simulink model "Model"  (R2020b)
settings: Solver=FixedStepAuto  StartTime=0.0  StopTime=12250  FixedStep=0.05  RelTol=1e-3
libraries: simulink x4
settings Model: Creator=Damerius  LastModifiedBy=Scythe
settings DataIOCC: ReturnWorkspaceOutputs=off
settings DebuggingCC: InheritedTsInSrcMsg=none  ArithmeticOperatorsInVariantConditions=warning
settings SFSimCC: SimUseLocalCustomCode=off  CustomCodeUndefinedFunction=UseInterfaceOnly
settings RTWCC: RTWUseLocalCustomCode=off

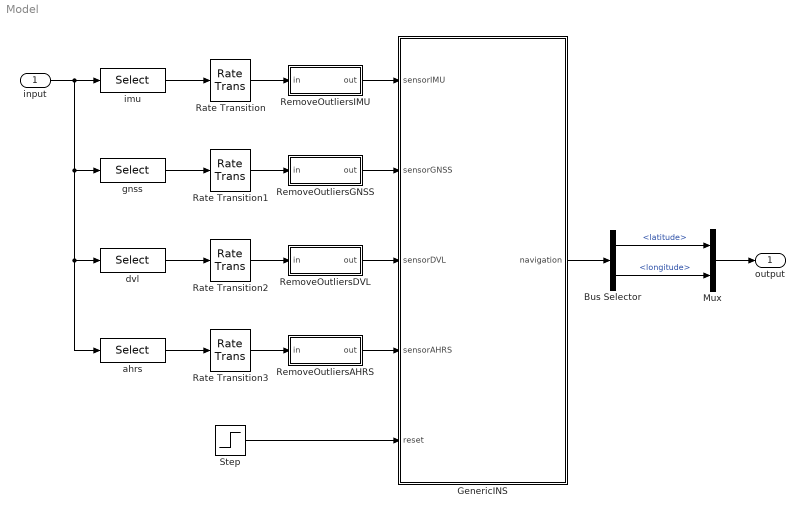
== system Model ==
  input : Inport
  Bus Selector : BusSelector  OutputSignals=latitude,longitude
  GenericINS : Subsystem
  Mux : Mux  Inputs=2
  Rate Transition{,1..3} (4 alike) : RateTransition  Integrity=off  Deterministic=off  OutPortSampleTime=0.05
  RemoveOutliersAHRS : Subsystem
  RemoveOutliersDVL : Subsystem
  RemoveOutliersGNSS : Subsystem
  RemoveOutliersIMU : Subsystem
  Step : Step  Time=0.05  Before=1  After=0
  ahrs : Selector  InputPortWidth=19  IndexOptions=Index vector (dialog)  Indices=16:19  OutputSizes=1
  dvl : Selector  InputPortWidth=19  IndexOptions=Index vector (dialog)  Indices=12:15  OutputSizes=1
  gnss : Selector  InputPortWidth=19  IndexOptions=Index vector (dialog)  Indices=8:11  OutputSizes=1
  imu : Selector  InputPortWidth=19  IndexOptions=Index vector (dialog)  Indices=1:7  OutputSizes=1
  output : Outport  VectorParamsAs1DForOutWhenUnconnected=off
  wires:
  input/1 -> imu/1, ahrs/1, dvl/1, gnss/1
  Mux/1 -> output/1
  Rate Transition1/1 -> RemoveOutliersGNSS/1(in)
  Rate Transition2/1 -> RemoveOutliersDVL/1(in)
  Rate Transition3/1 -> RemoveOutliersAHRS/1(in)
  imu/1 -> Rate Transition/1
  gnss/1 -> Rate Transition1/1
  dvl/1 -> Rate Transition2/1
  ahrs/1 -> Rate Transition3/1
  Rate Transition/1 -> RemoveOutliersIMU/1(in)
  RemoveOutliersIMU/1(out) -> GenericINS/1(sensorIMU)
  RemoveOutliersGNSS/1(out) -> GenericINS/2(sensorGNSS)
  RemoveOutliersDVL/1(out) -> GenericINS/3(sensorDVL)
  RemoveOutliersAHRS/1(out) -> GenericINS/4(sensorAHRS)
  GenericINS/1(navigation) -> Bus Selector/1
  Bus Selector/2 -> Mux/2  "<longitude>"
  Bus Selector/1 -> Mux/1  "<latitude>"
  Step/1 -> GenericINS/5(reset)

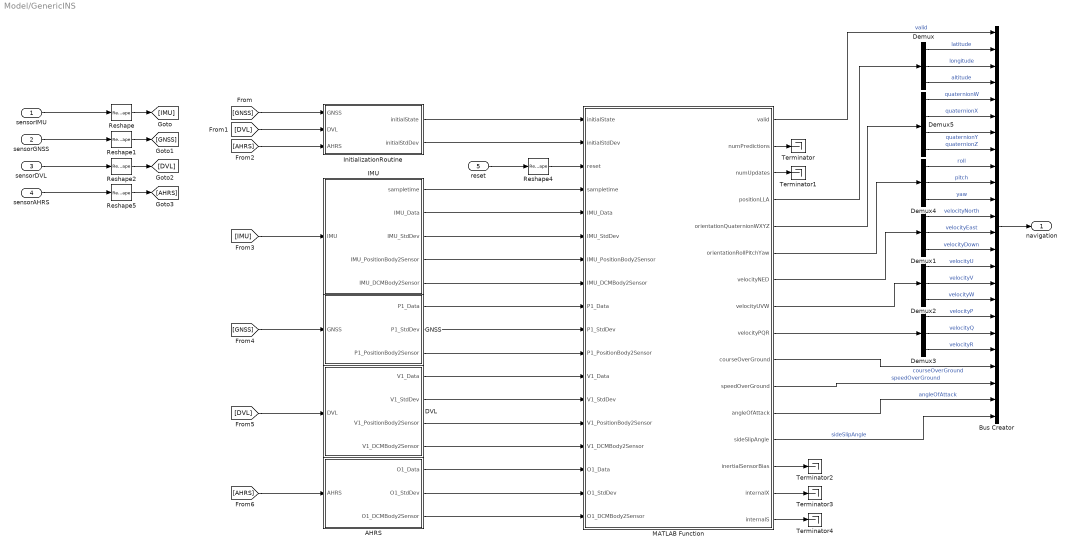
== system Model/GenericINS ==
  sensorIMU : Inport
  sensorGNSS : Inport  Port=2
  sensorDVL : Inport  Port=3
  sensorAHRS : Inport  Port=4
  reset : Inport  Port=5
  AHRS : Subsystem
  Bus Creator : BusCreator  Inputs=24
  DVL : Subsystem
  Demux{,1..4} (5 alike) : Demux  Outputs=3
  Demux5 : Demux
  GNSS : Subsystem
  IMU : Subsystem
  InitializationRoutine : Subsystem
  MATLAB Function : MATLAB Function  TreatAsAtomicUnit=on
  Reshape : Reshape  OutputDimensionality=Customize  OutputDimensions=[7,1]
  Reshape1 : Reshape  OutputDimensionality=Customize  OutputDimensions=[4,1]
  Reshape2 : Reshape  OutputDimensionality=Customize  OutputDimensions=[4,1]
  Reshape4 : Reshape  OutputDimensionality=Customize
  Reshape5 : Reshape  OutputDimensionality=Customize  OutputDimensions=[4,1]
  Terminator{,1..4} (5 alike) : Terminator
  navigation : Outport  VectorParamsAs1DForOutWhenUnconnected=off
  wires:
  Reshape5/1 -> [AHRS]
  sensorAHRS/1 -> Reshape5/1
  Reshape4/1 -> MATLAB Function/3(reset)
  reset/1 -> Reshape4/1
  Reshape2/1 -> [DVL]
  Reshape1/1 -> [GNSS]
  Reshape/1 -> [IMU]
  sensorGNSS/1 -> Reshape1/1
  sensorDVL/1 -> Reshape2/1
  sensorIMU/1 -> Reshape/1
  MATLAB Function/4(positionLLA) -> Demux/1
  MATLAB Function/7(velocityNED) -> Demux1/1
  MATLAB Function/8(velocityUVW) -> Demux2/1
  MATLAB Function/9(velocityPQR) -> Demux3/1
  MATLAB Function/5(orientationQuaternionWXYZ) -> Demux5/1
  Demux/1 -> Bus Creator/2  "latitude"
  Demux/2 -> Bus Creator/3  "longitude"
  Demux/3 -> Bus Creator/4  "altitude"
  Demux5/1 -> Bus Creator/5  "quaternionW"
  Demux5/2 -> Bus Creator/6  "quaternionX"
  Demux5/3 -> Bus Creator/7  "quaternionY"
  Demux5/4 -> Bus Creator/8  "quaternionZ"
  Demux4/1 -> Bus Creator/9  "roll"
  Demux4/2 -> Bus Creator/10  "pitch"
  Demux4/3 -> Bus Creator/11  "yaw"
  Demux1/1 -> Bus Creator/12  "velocityNorth"
  Demux1/2 -> Bus Creator/13  "velocityEast"
  Demux1/3 -> Bus Creator/14  "velocityDown"
  Demux2/1 -> Bus Creator/15  "velocityU"
  Demux2/2 -> Bus Creator/16  "velocityV"
  Demux2/3 -> Bus Creator/17  "velocityW"
  Demux3/1 -> Bus Creator/18  "velocityP"
  Demux3/2 -> Bus Creator/19  "velocityQ"
  Demux3/3 -> Bus Creator/20  "velocityR"
  Bus Creator/1 -> navigation/1
  InitializationRoutine/1(initialState) -> MATLAB Function/1(initialState)
  InitializationRoutine/2(initialStdDev) -> MATLAB Function/2(initialStdDev)
  [GNSS] -> InitializationRoutine/1(GNSS)
  [DVL] -> InitializationRoutine/2(DVL)
  [AHRS] -> InitializationRoutine/3(AHRS)
  [IMU] -> IMU/1(IMU)
  IMU/1(sampletime) -> MATLAB Function/4(sampletime)
  IMU/2(IMU_Data) -> MATLAB Function/5(IMU_Data)
  IMU/4(IMU_PositionBody2Sensor) -> MATLAB Function/7(IMU_PositionBody2Sensor)
  IMU/5(IMU_DCMBody2Sensor) -> MATLAB Function/8(IMU_DCMBody2Sensor)
  GNSS/3(P1_PositionBody2Sensor) -> MATLAB Function/11(P1_PositionBody2Sensor)
  [GNSS] -> GNSS/1(GNSS)
  DVL/3(V1_PositionBody2Sensor) -> MATLAB Function/14(V1_PositionBody2Sensor)
  DVL/4(V1_DCMBody2Sensor) -> MATLAB Function/15(V1_DCMBody2Sensor)
  [DVL] -> DVL/1(DVL)
  AHRS/3(O1_DCMBody2Sensor) -> MATLAB Function/18(O1_DCMBody2Sensor)
  [AHRS] -> AHRS/1(AHRS)
  MATLAB Function/6(orientationRollPitchYaw) -> Demux4/1
  MATLAB Function/1(valid) -> Bus Creator/1  "valid"
  MATLAB Function/10(courseOverGround) -> Bus Creator/21  "courseOverGround"
  MATLAB Function/11(speedOverGround) -> Bus Creator/22  "speedOverGround"
  MATLAB Function/12(angleOfAttack) -> Bus Creator/23  "angleOfAttack"
  MATLAB Function/13(sideSlipAngle) -> Bus Creator/24  "sideSlipAngle"
  AHRS/1(O1_Data) -> MATLAB Function/16(O1_Data)
  AHRS/2(O1_StdDev) -> MATLAB Function/17(O1_StdDev)
  DVL/2(V1_StdDev) -> MATLAB Function/13(V1_StdDev)
  GNSS/1(P1_Data) -> MATLAB Function/9(P1_Data)
  GNSS/2(P1_StdDev) -> MATLAB Function/10(P1_StdDev)
  IMU/3(IMU_StdDev) -> MATLAB Function/6(IMU_StdDev)
  DVL/1(V1_Data) -> MATLAB Function/12(V1_Data)
  MATLAB Function/2(numPredictions) -> Terminator/1
  MATLAB Function/3(numUpdates) -> Terminator1/1
  MATLAB Function/14(inertialSensorBias) -> Terminator2/1
  MATLAB Function/15(internalX) -> Terminator3/1
  MATLAB Function/16(internalS) -> Terminator4/1

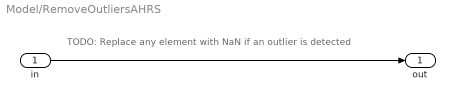
== system Model/RemoveOutliersAHRS ==
  note: TODO: Replace any element with NaN if an outlier is detected
  in : Inport
  out : Outport  VectorParamsAs1DForOutWhenUnconnected=off
  wires:
  in/1 -> out/1

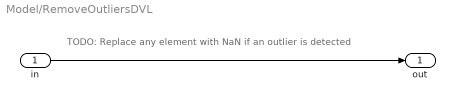
== system Model/RemoveOutliersDVL ==
  note: TODO: Replace any element with NaN if an outlier is detected
  in : Inport
  out : Outport  VectorParamsAs1DForOutWhenUnconnected=off
  wires:
  in/1 -> out/1

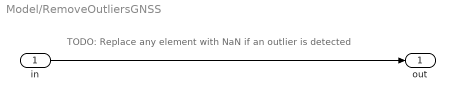
== system Model/RemoveOutliersGNSS ==
  note: TODO: Replace any element with NaN if an outlier is detected
  in : Inport
  out : Outport  VectorParamsAs1DForOutWhenUnconnected=off
  wires:
  in/1 -> out/1

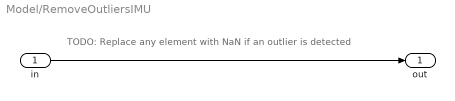
== system Model/RemoveOutliersIMU ==
  note: TODO: Replace any element with NaN if an outlier is detected
  in : Inport
  out : Outport  VectorParamsAs1DForOutWhenUnconnected=off
  wires:
  in/1 -> out/1

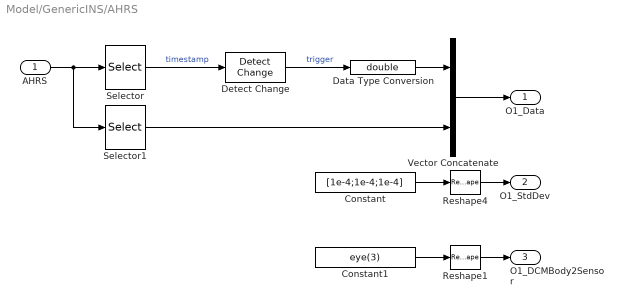
== system Model/GenericINS/AHRS ==
  AHRS : Inport
  Constant : Constant  Value=[1e-4;1e-4;1e-4]
  Constant1 : Constant  Value=eye(3)
  Data Type Conversion : DataTypeConversion  OutDataTypeStr=double
  Detect Change : simulink/Logic and Bit Operations/Detect Change  vinit=0  OutDataTypeStr=boolean
  Reshape1 : Reshape  OutputDimensionality=Customize  OutputDimensions=[3,3]
  Reshape4 : Reshape  OutputDimensionality=Customize  OutputDimensions=[3,1]
  Selector : Selector  InputPortWidth=4  IndexOptions=Index vector (dialog)  Indices=1  OutputSizes=1
  Selector1 : Selector  InputPortWidth=4  IndexOptions=Index vector (dialog)  Indices=2:4  OutputSizes=1
  Vector Concatenate : Concatenate
  O1_Data : Outport  VectorParamsAs1DForOutWhenUnconnected=off
  O1_StdDev : Outport  Port=2  VectorParamsAs1DForOutWhenUnconnected=off
  O1_DCMBody2Sensor : Outport  Port=3  VectorParamsAs1DForOutWhenUnconnected=off
  wires:
  Constant1/1 -> Reshape1/1
  Constant/1 -> Reshape4/1
  Vector Concatenate/1 -> O1_Data/1
  Selector1/1 -> Vector Concatenate/2
  Data Type Conversion/1 -> Vector Concatenate/1
  Detect Change/1 -> Data Type Conversion/1  "trigger"
  Selector/1 -> Detect Change/1  "timestamp"
  AHRS/1 -> Selector/1, Selector1/1
  Reshape4/1 -> O1_StdDev/1
  Reshape1/1 -> O1_DCMBody2Sensor/1

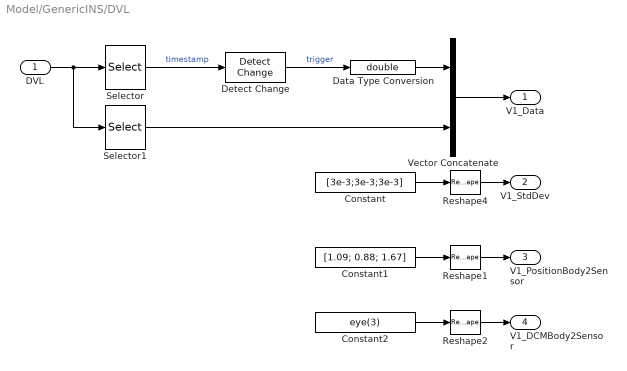
== system Model/GenericINS/DVL ==
  DVL : Inport
  Constant : Constant  Value=[3e-3;3e-3;3e-3]
  Constant1 : Constant  Value=[1.09; 0.88; 1.67]
  Constant2 : Constant  Value=eye(3)
  Data Type Conversion : DataTypeConversion  OutDataTypeStr=double
  Detect Change : simulink/Logic and Bit Operations/Detect Change  vinit=0  OutDataTypeStr=boolean
  Reshape1 : Reshape  OutputDimensionality=Customize  OutputDimensions=[3,1]
  Reshape2 : Reshape  OutputDimensionality=Customize  OutputDimensions=[3,3]
  Reshape4 : Reshape  OutputDimensionality=Customize  OutputDimensions=[3,1]
  Selector : Selector  InputPortWidth=4  IndexOptions=Index vector (dialog)  Indices=1  OutputSizes=1
  Selector1 : Selector  InputPortWidth=4  IndexOptions=Index vector (dialog)  Indices=2:4  OutputSizes=1
  Vector Concatenate : Concatenate
  V1_Data : Outport  VectorParamsAs1DForOutWhenUnconnected=off
  V1_StdDev : Outport  Port=2  VectorParamsAs1DForOutWhenUnconnected=off
  V1_PositionBody2Sensor : Outport  Port=3  VectorParamsAs1DForOutWhenUnconnected=off
  V1_DCMBody2Sensor : Outport  Port=4  VectorParamsAs1DForOutWhenUnconnected=off
  wires:
  Constant1/1 -> Reshape1/1
  Constant/1 -> Reshape4/1
  Vector Concatenate/1 -> V1_Data/1
  Selector1/1 -> Vector Concatenate/2
  Data Type Conversion/1 -> Vector Concatenate/1
  Detect Change/1 -> Data Type Conversion/1  "trigger"
  Selector/1 -> Detect Change/1  "timestamp"
  DVL/1 -> Selector/1, Selector1/1
  Constant2/1 -> Reshape2/1
  Reshape4/1 -> V1_StdDev/1
  Reshape1/1 -> V1_PositionBody2Sensor/1
  Reshape2/1 -> V1_DCMBody2Sensor/1

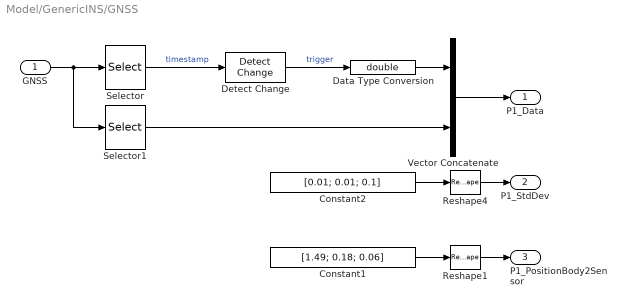
== system Model/GenericINS/GNSS ==
  GNSS : Inport
  Constant1 : Constant  Value=[1.49; 0.18; 0.06]
  Constant2 : Constant  Value=[0.01; 0.01; 0.1]
  Data Type Conversion : DataTypeConversion  OutDataTypeStr=double
  Detect Change : simulink/Logic and Bit Operations/Detect Change  vinit=0  OutDataTypeStr=boolean
  Reshape1 : Reshape  OutputDimensionality=Customize  OutputDimensions=[3,1]
  Reshape4 : Reshape  OutputDimensionality=Customize  OutputDimensions=[3,1]
  Selector : Selector  InputPortWidth=4  IndexOptions=Index vector (dialog)  Indices=1  OutputSizes=1
  Selector1 : Selector  InputPortWidth=4  IndexOptions=Index vector (dialog)  Indices=2:4  OutputSizes=1
  Vector Concatenate : Concatenate
  P1_Data : Outport  VectorParamsAs1DForOutWhenUnconnected=off
  P1_StdDev : Outport  Port=2  VectorParamsAs1DForOutWhenUnconnected=off
  P1_PositionBody2Sensor : Outport  Port=3  VectorParamsAs1DForOutWhenUnconnected=off
  wires:
  GNSS/1 -> Selector1/1, Selector/1
  Selector/1 -> Detect Change/1  "timestamp"
  Detect Change/1 -> Data Type Conversion/1  "trigger"
  Data Type Conversion/1 -> Vector Concatenate/1
  Selector1/1 -> Vector Concatenate/2
  Vector Concatenate/1 -> P1_Data/1
  Constant2/1 -> Reshape4/1
  Constant1/1 -> Reshape1/1
  Reshape4/1 -> P1_StdDev/1
  Reshape1/1 -> P1_PositionBody2Sensor/1

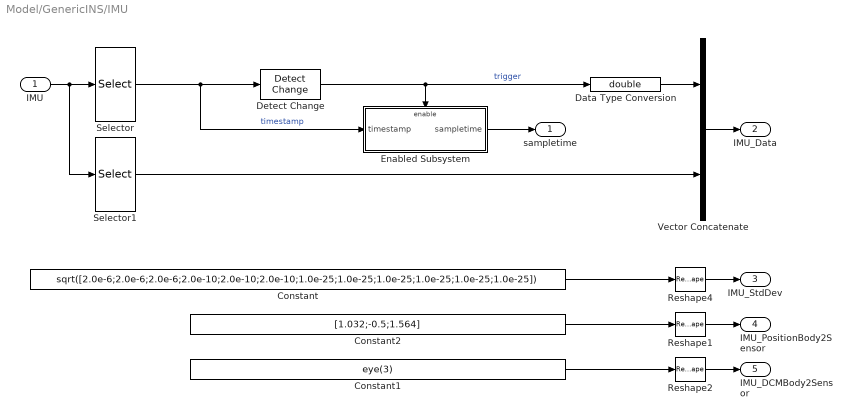
== system Model/GenericINS/IMU ==
  IMU : Inport
  Constant : Constant  Value=sqrt([2.0e-6;2.0e-6;2.0e-6;2.0e-10;2.0e-10;2.0e-10;1.0e-25;1.0e-25;1.0e-25;1.0e-25;1.0e-25;1.0e-25])
  Constant1 : Constant  Value=eye(3)
  Constant2 : Constant  Value=[1.032;-0.5;1.564]
  Data Type Conversion : DataTypeConversion  OutDataTypeStr=double
  Detect Change : simulink/Logic and Bit Operations/Detect Change  vinit=0  OutDataTypeStr=boolean
  Enabled Subsystem : Subsystem  TreatAsAtomicUnit=on
  Reshape1 : Reshape  OutputDimensionality=Customize  OutputDimensions=[3,1]
  Reshape2 : Reshape  OutputDimensionality=Customize  OutputDimensions=[3,3]
  Reshape4 : Reshape  OutputDimensionality=Customize  OutputDimensions=[12,1]
  Selector : Selector  InputPortWidth=7  IndexOptions=Index vector (dialog)  Indices=1  OutputSizes=1
  Selector1 : Selector  InputPortWidth=7  IndexOptions=Index vector (dialog)  Indices=2:7  OutputSizes=1
  Vector Concatenate : Concatenate
  sampletime : Outport  VectorParamsAs1DForOutWhenUnconnected=off
  IMU_Data : Outport  Port=2  VectorParamsAs1DForOutWhenUnconnected=off
  IMU_StdDev : Outport  Port=3  VectorParamsAs1DForOutWhenUnconnected=off
  IMU_PositionBody2Sensor : Outport  Port=4  VectorParamsAs1DForOutWhenUnconnected=off
  IMU_DCMBody2Sensor : Outport  Port=5  VectorParamsAs1DForOutWhenUnconnected=off
  wires:
  Constant/1 -> Reshape4/1
  Constant1/1 -> Reshape2/1
  Constant2/1 -> Reshape1/1
  Selector/1 -> Enabled Subsystem/1(timestamp), Detect Change/1  "timestamp"
  Detect Change/1 -> Enabled Subsystem/Enable, Data Type Conversion/1  "trigger"
  Enabled Subsystem/1(sampletime) -> sampletime/1
  Data Type Conversion/1 -> Vector Concatenate/1
  IMU/1 -> Selector1/1, Selector/1
  Selector1/1 -> Vector Concatenate/2
  Vector Concatenate/1 -> IMU_Data/1
  Reshape4/1 -> IMU_StdDev/1
  Reshape1/1 -> IMU_PositionBody2Sensor/1
  Reshape2/1 -> IMU_DCMBody2Sensor/1

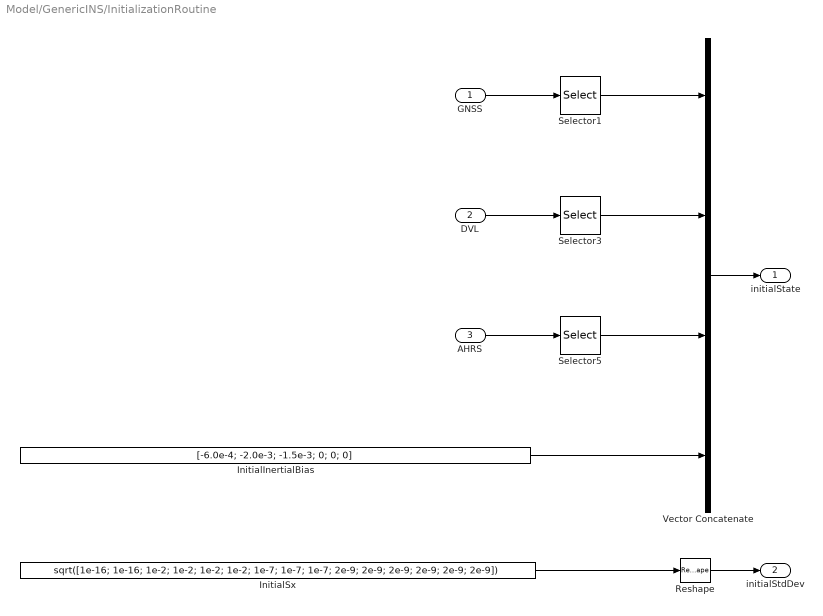
== system Model/GenericINS/InitializationRoutine ==
  GNSS : Inport
  DVL : Inport  Port=2
  AHRS : Inport  Port=3
  InitialInertialBias : Constant  Value=[-6.0e-4; -2.0e-3; -1.5e-3; 0; 0; 0]
  InitialSx : Constant  Value=sqrt([1e-16; 1e-16; 1e-2; 1e-2; 1e-2; 1e-2; 1e-7; 1e-7; 1e-7; 2e-9; 2e-9; 2e-9; 2e-9; 2e-9; 2e-9])
  Reshape : Reshape  OutputDimensionality=Customize  OutputDimensions=[15,1]
  Selector1 : Selector  InputPortWidth=4  IndexOptions=Index vector (dialog)  Indices=2:4  OutputSizes=1
  Selector3 : Selector  InputPortWidth=4  IndexOptions=Index vector (dialog)  Indices=2:4  OutputSizes=1
  Selector5 : Selector  InputPortWidth=4  IndexOptions=Index vector (dialog)  Indices=2:4  OutputSizes=1
  Vector Concatenate : Concatenate  NumInputs=4
  initialState : Outport  VectorParamsAs1DForOutWhenUnconnected=off
  initialStdDev : Outport  Port=2  VectorParamsAs1DForOutWhenUnconnected=off
  wires:
  Selector1/1 -> Vector Concatenate/1
  GNSS/1 -> Selector1/1
  DVL/1 -> Selector3/1
  Selector3/1 -> Vector Concatenate/2
  Selector5/1 -> Vector Concatenate/3
  AHRS/1 -> Selector5/1
  InitialInertialBias/1 -> Vector Concatenate/4
  Vector Concatenate/1 -> initialState/1
  Reshape/1 -> initialStdDev/1
  InitialSx/1 -> Reshape/1

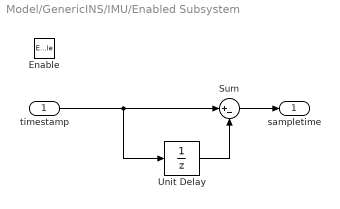
== system Model/GenericINS/IMU/Enabled Subsystem ==
  timestamp : Inport
  Enable : EnablePort
  Sum : Sum  Inputs=|+-
  Unit Delay : UnitDelay  SampleTime=-1  HasFrameUpgradeWarning=on
  sampletime : Outport  VectorParamsAs1DForOutWhenUnconnected=off
  wires:
  timestamp/1 -> Unit Delay/1, Sum/1
  Unit Delay/1 -> Sum/2
  Sum/1 -> sampletime/1

== matlab function Model/GenericINS/MATLAB Function ==
  data: initialState input; valid output; numPredictions output; numUpdates output; initialStdDev input; reset input; sampletime input; IMU_Data input; IMU_StdDev input; IMU_PositionBody2Sensor input; IMU_DCMBody2Sensor input; P1_Data input; P1_StdDev input; P1_PositionBody2Sensor input; V1_Data input; V1_StdDev input; V1_PositionBody2Sensor input; V1_DCMBody2Sensor input; O1_Data input; O1_StdDev input; O1_DCMBody2Sensor input; positionLLA output; orientationQuaternionWXYZ output; orientationRollPitchYaw output; velocityNED output; velocityUVW output; velocityPQR output; courseOverGround output; speedOverGround output; angleOfAttack output; sideSlipAngle output; inertialSensorBias output; internalX output; internalS output
function [valid, numPredictions, numUpdates, positionLLA, orientationQuaternionWXYZ, orientationRollPitchYaw, velocityNED, velocityUVW, velocityPQR, courseOverGround, speedOverGround, angleOfAttack, sideSlipAngle, inertialSensorBias, internalX, internalS] = ExampleINS(initialState, initialStdDev, reset, sampletime, IMU_Data, IMU_StdDev, IMU_PositionBody2Sensor, IMU_DCMBody2Sensor, P1_Data, P1_StdDev, P1_PositionBody2Sensor, V1_Data, V1_StdDev, V1_PositionBody2Sensor, V1_DCMBody2Sensor, O1_Data, O1_StdDev, O1_DCMBody2Sensor)
    %ExampleINS Generated MATLAB function for a generic inertial navigation system (1 position measurements, 1 velocity measurements, 1 orientation measurements).
    % This function was automatically generated using the command GenericINS.GenerateFunction('ExampleINS', [3], [3], [3], 0).
    % 
    % PARAMETERS
    % initialState               ... 15-by-1 initial state vector to be used when the INS is reset. The elements are as follows:
    %                                 1: latitude     [rad]     Initial latitude of the position of the IMU.
    %                                 2: longitude    [rad]     Initial longitude of the position of the IMU.
    %                                 3: altitude     [m]       Initial altitude of the position of the IMU, positive upwards.
    %                                 4: velocityU    [m/s]     Initial body-fixed velocity in x-direction of the body-frame at the position of the IMU.
    %                                 5: velocityV    [m/s]     Initial body-fixed velocity in y-direction of the body-frame at the position of the IMU.
    %                                 6: velocityW    [m/s]     Initial body-fixed velocity in z-direction of the body-frame at the position of the IMU.
    %                                 7: roll         [rad]     Initial roll angle.
    %                                 8: pitch        [rad]     Initial pitch angle.
    %                                 9: yaw          [rad]     Initial yaw angle.
    %                                10: biasAccX     [m/(s*s)] Initial acceleration bias in x-direction of IMU sensor frame.
    %                                11: biasAccY     [m/(s*s)] Initial acceleration bias in y-direction of IMU sensor frame.
    %                                12: biasAccZ     [m/(s*s)] Initial acceleration bias in z-direction of IMU sensor frame.
    %                                13: biasGyrX     [rad/s]   Initial angular rate bias around x-axis of IMU sensor frame.
    %                                14: biasGyrY     [rad/s]   Initial angular rate bias around y-axis of IMU sensor frame.
    %                                15: biasGyrZ     [rad/s]   Initial angular rate bias around z-axis of IMU sensor frame.
    % initialStdDev              ... 15-by-1 standard deviation vector that represents the unvertainty of the initial state. It is better to use larger values than
    %                                too small values for the filter to converge. The elements are as follows:
    %                                 1: latitude     [rad]     Initial standard deviation for initial latitude.
    %                                 2: longitude    [rad]     Initial standard deviation for initial longitude.
    %                                 3: altitude     [m]       Initial standard deviation for initial altitude.
    %                                 4: velocityU    [m/s]     Initial standard deviation for initial body-fixed velocity in x-direction of the body-frame.
    %                                 5: velocityV    [m/s]     Initial standard deviation for initial body-fixed velocity in y-direction of the body-frame.
    %                                 6: velocityW    [m/s]     Initial standard deviation for initial body-fixed velocity in z-direction of the body-frame.
    %                                 7: orientationX           Initial standard deviation for x-component of orientation vector (axis-angle representation).
    %                                 8: orientationY           Initial standard deviation for y-component of orientation vector (axis-angle representation).
    %                                 9: orientationZ           Initial standard deviation for z-component of orientation vector (axis-angle representation).
    %                                10: biasAccX     [m/(s*s)] Initial standard deviation for acceleration bias in x-direction of IMU sensor frame.
    %                                11: biasAccY     [m/(s*s)] Initial standard deviation for acceleration bias in y-direction of IMU sensor frame.
    %                                12: biasAccZ     [m/(s*s)] Initial standard deviation for acceleration bias in z-direction of IMU sensor frame.
    %                                13: biasGyrX     [rad/s]   Initial standard deviation for angular rate bias around x-axis of IMU sensor frame.
    %                                14: biasGyrY     [rad/s]   Initial standard deviation for angular rate bias around y-axis of IMU sensor frame.
    %                                15: biasGyrZ     [rad/s]   Initial standard deviation for angular rate bias around z-axis of IMU sensor frame.
    % reset                      ... Greater than 0.0 if filter should be reset/reinitialized, 0.0 otherwise. During an initialization the initial state and initial standard deviations are used.
    % sampletime                 ... Discrete sampletime in seconds to be used for forward euler integration. Should be the elapsed time to the latest prediction.
    % IMU_Data                   ... The 7-by-1 vector representing the IMU data where the elements are as follows:
    %                                 1: trigger                Greater than 0.0 if new IMU data is available and should be used in a prediction step, 0.0 otherwise.
    %                                 2: accX         [m/(s*s)] Acceleration in x-direction of IMU sensor frame.
    %                                 3: accY         [m/(s*s)] Acceleration in y-direction of IMU sensor frame.
    %                                 4: accZ         [m/(s*s)] Acceleration in z-direction of IMU sensor frame.
    %                                 5: gyrX         [rad/s]   Angular rate around x-axis of IMU sensor frame.
    %                                 6: gyrY         [rad/s]   Angular rate around y-axis of IMU sensor frame.
    %                                 7: gyrZ         [rad/s]   Angular rate around z-axis of IMU sensor frame.
    % IMU_StdDev                 ... 12-by-1 vector representing the standard deviation for inertial measurements and inertial biases. The elements are as follows:
    %                                 1: accX         [m/(s*s)] Standard deviation for acceleration in x-direction of IMU sensor frame.
    %                                 2: accY         [m/(s*s)] Standard deviation for acceleration in y-direction of IMU sensor frame.
    %                                 3: accZ         [m/(s*s)] Standard deviation for acceleration in z-direction of IMU sensor frame.
    %                                 4: gyrX         [rad/s]   Standard deviation for angular rate around x-axis of IMU sensor frame.
    %                                 5: gyrY         [rad/s]   Standard deviation for angular rate around y-axis of IMU sensor frame.
    %                                    6: gyrZ         [rad/s]   Standard deviation for angular rate around z-axis of IMU sensor frame.
    %                                 7: biasAccX     [m/(s*s)] Standard deviation for acceleration bias in x-direction of IMU sensor frame.
    %                                 8: biasAccY     [m/(s*s)] Standard deviation for acceleration bias in y-direction of IMU sensor frame.
    %                                 9: biasAccZ     [m/(s*s)] Standard deviation for acceleration bias in z-direction of IMU sensor frame.
    %                                10: biasGyrX     [rad/s]   Standard deviation for angular rate bias around x-axis of IMU sensor frame.
    %                                11: biasGyrY     [rad/s]   Standard deviation for angular rate bias around y-axis of IMU sensor frame.
    %                                12: biasGyrZ     [rad/s]   Standard deviation for angular rate bias around z-axis of IMU sensor frame.
    % IMU_PositionBody2Sensor    ... Position of IMU sensor frame origin w.r.t. body frame origin in body frame coordinates (meters).
    % IMU_DCMBody2Sensor         ... Direction cosine matrix to rotate measurements from body frame to sensor frame.
    % P1_Data                    ... 4-by-1 vector representing the position measurements of position sensor 1. The elements are as follows:
    %                                 1: trigger                Greater than 0.0 if new measurement data is available and should be used in an update step, 0.0 otherwise.
    %                                 2: latitude     [rad]     The latitude measurement.
    %                                 3: longitude    [rad]     The longitude measurement.
    %                                 4: altitude     [m]       The altitude measurement.
    % P1_StdDev                  ... 3-by-1 vector representing the standard deviation for the position measurements of position sensor 1. The elements are as follows:
    %                                 1: stdNorth     [m]       Standard deviation in north direction.
    %                                 2: stdEast      [m]       Standard deviation in east direction.
    %                                 3: stdDown      [m]       Standard deviation in up/down-direction.
    % P1_PositionBody2Sensor     ... Position of position sensor 1 w.r.t. body frame origin in body frame coordinates (meters).
    % V1_Data                    ... 4-by-1 vector representing the velocity measurements of velocity sensor 1. The elements are as follows:
    %                                 1: trigger                Greater than 0.0 if new measurement data is available and should be used in an update step, 0.0 otherwise.
    %                                 2: velocityX    [m/s]     The velocity measurement in x-direction of sensor frame.
    %                                 3: velocityY    [m/s]     The velocity measurement in y-direction of sensor frame.
    %                                 4: velocityZ    [m/s]     The velocity measurement in z-direction of sensor frame.
    % V1_StdDev                  ... 3-by-1 vector representing the standard deviation for the velocity measurements of velocity sensor 1. The elements are as follows:
    %                                 1: stdX         [m/s]     Standard deviation in x-direction.
    %                                 2: stdY         [m/s]     Standard deviation in y-direction.
    %                                 3: stdZ         [m/s]     Standard deviation in z-direction.
    % V1_PositionBody2Sensor     ... Position of velocity sensor 1 w.r.t. body frame origin in body frame coordinates (meters).
    % V1_DCMBody2Sensor          ... Direction cosine matrix to rotate vectors from body frame to sensor frame.
    % O1_Data                    ... 4-by-1 vector representing the orientation measurements of orientation sensor 1. Note that orientation measurements must only be used for applications with small roll and pitch angles. The elements are as follows:
    %                                 1: trigger                Greater than 0.0 if new measurement data is available and should be used in an update step, 0.0 otherwise.
    %                                 2: roll         [rad]     The roll angle measurement (ZYX-convention).
    %                                 3: pitch        [rad]     The pitch angle measurement (ZYX-convention).
    %                                 4: yaw          [rad]     The yaw angle measurement (ZYX-convention).
    % O1_StdDev                  ... 3-by-1 vector representing the standard deviation for the orientation measurements of orientation sensor 1. The elements are as follows:
    %                                 1: stdRoll      [rad]     Standard deviation for roll angle.
    %                                 2: stdPitch     [rad]     Standard deviation for pitch angle.
    %                                 3: stdYaw       [rad]     Standard deviation for yaw angle.
    % O1_DCMBody2Sensor          ... Direction cosine matrix to rotate vectors from body frame to sensor frame.
    % 
    % RETURN
    % valid                      ... A scalar boolean that indicates whether the motion state is valid or not. It is valid if the INS was initialized.
    % numPredictions             ... An integer indicating the number of prediction steps that have been calculated (either 0 or 1).
    % numUpdates                 ... An integer indicating the number of update steps that have been calculated.
    % positionLLA                ... Geographic position of the body frame, [lat (rad); lon (rad); alt (m, positive upwards)].
    % orientationQuaternionWXYZ  ... Unit quaternion describing a rotation from body frame to navigation frame, [qw; qx; qy; qz], where qw indicates the scalar part of the quaternion.
    % orientationRollPitchYaw    ... Euler angles according to the ZYX-convention.
    % velocityNED                ... Translational velocity [m/s] of the body frame given in navigation frame coordinates, excluding earth rotation and transport rate.
    % velocityUVW                ... Translational velocity [m/s] of the body frame given in body frame coordinates, excluding earth rotation and transport rate.
    % velocityPQR                ... Rotational velocity [rad/s] of the body frame with respect to the navigation frame, excluding earth rotation and transport rate.
    % courseOverGround           ... Course over ground angle in radians.
    % speedOverGround            ... Speed over ground in meters per second.
    % angleOfAttack              ... Angle of attack in radians.
    % sideSlipAngle              ... Side slip angle in radians.
    % inertialSensorBias         ... Inertial sensor bias [accX (m/s^2); accY (m/s^2); accZ (m/s^2); gyrX (rad/s); gyrY (rad/s); gyrZ (rad/s)].
    % internalX                  ... 16-by-1 state vector representing the internal motion state with respect to the IMU. Elements are as follows:
    %                            ...  1: Latitude in radians.
    %                            ...  2: Longitude in radians.
    %                            ...  3: Altitude in meters (positive upwards).
    %                            ...  4: North velocity in meters per second.
    %                            ...  5: East velocity in meters per second.
    %                            ...  6: Down velocity in meters per second.
    %                            ...  7: Scalar part of unit quaternion.
    %                            ...  8: First element of vector part of unit quaternion.
    %                            ...  9: Second element of vector part of unit quaternion.
    %                            ... 10: Third element of vector part of unit quaternion.
    %                            ... 11: Accelerometer bias (x) in m/s^2.
    %                            ... 12: Accelerometer bias (y) in m/s^2.
    %                            ... 13: Accelerometer bias (z) in m/s^2.
    %                            ... 14: Gyroscope bias (x) in rad/s.
    %                            ... 15: Gyroscope bias (x) in rad/s.
    %                            ... 16: Gyroscope bias (x) in rad/s.
    % internalS                  ... 15-by-15 matrix representing the internal square root of the state covariance matrix. This matrix relates to the internalX state. Note that the uncertainty of the quaternion (4D) is represented by an orientation vector (3D).
    assert((15 == size(initialState,1)) && (1 == size(initialState,2)) && (15 == size(initialStdDev,1)) && (1 == size(initialStdDev,2)) && isscalar(reset) && isscalar(sampletime) && (7 == size(IMU_Data,1)) && (1 == size(IMU_Data,2)) && (3 == size(IMU_PositionBody2Sensor,1)) && (1 == size(IMU_PositionBody2Sensor,2)) && (3 == size(IMU_DCMBody2Sensor,1)) && (3 == size(IMU_DCMBody2Sensor,2)));
    persistent ins; if(isempty(ins)), ins = GenericINS(); end
    persistent imuStdDevBuffer; if(isempty(imuStdDevBuffer)), imuStdDevBuffer = IMU_StdDev; end

    assert((4 == size(P1_Data,1)) && (1 == size(P1_Data,2)) && (3 == size(P1_StdDev,1)) && (1 == size(P1_StdDev,2)) && (3 == size(P1_PositionBody2Sensor,1)) && (1 == size(P1_PositionBody2Sensor,2)));
    persistent P1_Buffer; if(isempty(P1_Buffer) || (P1_Data(1) > 0.0)), P1_Buffer = P1_Data; end
    assert((4 == size(V1_Data,1)) && (1 == size(V1_Data,2)) && (3 == size(V1_StdDev,1)) && (1 == size(V1_StdDev,2)) && (3 == size(V1_PositionBody2Sensor,1)) && (1 == size(V1_PositionBody2Sensor,2)) && (3 == size(V1_DCMBody2Sensor,1)) && (3 == size(V1_DCMBody2Sensor,2)));
    persistent V1_Buffer; if(isempty(V1_Buffer) || (V1_Data(1) > 0.0)), V1_Buffer = V1_Data; end
    assert((4 == size(O1_Data,1)) && (1 == size(O1_Data,2)) && (3 == size(O1_StdDev,1)) && (1 == size(O1_StdDev,2)) && (3 == size(O1_DCMBody2Sensor,1)) && (3 == size(O1_DCMBody2Sensor,2)));
    persistent O1_Buffer; if(isempty(O1_Buffer) || (O1_Data(1) > 0.0)), O1_Buffer = O1_Data; end

    imuStdDevChanged = (sum(abs(imuStdDevBuffer - IMU_StdDev) > 100*eps) > 0.0);
    if(reset > 0.0)
        ins.Initialize(initialState(1:3), initialState(4:6), initialState(7:9), initialState(10:12), initialState(13:15), initialStdDev(1:3), initialStdDev(4:6), initialStdDev(7:9), initialStdDev(10:12), initialStdDev(13:15), IMU_StdDev(1:3), IMU_StdDev(4:6), IMU_StdDev(7:9), IMU_StdDev(10:12));
    elseif(imuStdDevChanged)
        ins.ResetInertialStandardDeviation(IMU_StdDev(1:3), IMU_StdDev(4:6), IMU_StdDev(7:9), IMU_StdDev(10:12));
    end
    imuStdDevBuffer = IMU_StdDev;
    numPredictions = int32(0);
    numUpdates = int32(0);
    if(IMU_Data(1) > 0.0)
        % Motion prediction
        numPredictions = int32(1);
        ins.Predict(IMU_Data(2:7), sampletime, IMU_DCMBody2Sensor, IMU_PositionBody2Sensor);

        % Sensor updates
        if(P1_Buffer(1) > 0.0), numUpdates = numUpdates + int32(1); P1_Buffer(1) = 0.0; ins.UpdatePosition3D(P1_Buffer(2:end), P1_StdDev, P1_PositionBody2Sensor); end
        if(V1_Buffer(1) > 0.0), numUpdates = numUpdates + int32(1); V1_Buffer(1) = 0.0; ins.UpdateVelocity3D(V1_Buffer(2:end), V1_StdDev, V1_PositionBody2Sensor, V1_DCMBody2Sensor); end
        if(O1_Buffer(1) > 0.0), numUpdates = numUpdates + int32(1); O1_Buffer(1) = 0.0; ins.UpdateOrientation3D(O1_Buffer(2:end), O1_StdDev, O1_DCMBody2Sensor); end
    end
    [valid, positionLLA, orientationQuaternionWXYZ, orientationRollPitchYaw, velocityNED, velocityUVW, velocityPQR, courseOverGround, speedOverGround, angleOfAttack, sideSlipAngle, inertialSensorBias] = ins.GetMotionState();
    [internalX, internalS] = ins.GetInternalState();
end
